simulink library "mlepLibrary"  (R2018a)
settings: Solver=ode45  StartTime=0.0  StopTime=10.0  RelTol=1e-3
undefined symbols (not defined in the file or in its folder): cs_val
settings Model: Creator=willyg  LastModifiedBy=E592090
settings DataIOCC: LimitDataPoints=on  SaveFormat=Array  SignalLoggingSaveFormat=ModelDataLogs
settings OptimizationCC: BlockReduction=off  BooleanDataType=off  LifeSpan=inf
settings DebuggingCC: SaveWithParameterizedLinksMsg=none  UnderspecifiedInitializationDetection=Classic  MergeDetectMultiDrivingBlocksExec=none  SignalResolutionControl=TryResolveAllWithWarning  MultiTaskDSMMsg=warning  MultiTaskCondExecSysMsg=none  SFUnexpectedBacktrackingDiag=warning  SFNoUnconditionalDefaultTransitionDiag=warning  SFExecutionAtInitializationDiag=none
settings HardwareCC: ProdBitPerPointer=32  ProdBitPerSizeT=32  ProdBitPerPtrDiffT=32  ProdLargestAtomicFloat=None  ProdIntDivRoundTo=Undefined  ProdEndianess=Unspecified  ProdWordSize=32  ProdHWDeviceType=32-bit Generic  TargetUnknown=on
settings ModelReferenceCC: PropagateSignalLabelsOutOfModel=off
settings CodeAppCC: StateflowObjectComments=on
settings GRTTargetCC: TargetLangStandard=C89/C90 (ANSI)  GeneratePreprocessorConditionals=Disable all
settings ConfigComp: CovMetricSettings=dw  CovHtmlReporting=on  CovSaveCumulativeToWorkspaceVar=on  CovSaveSingleToWorkspaceVar=on  CovExternalEMLEnable=off

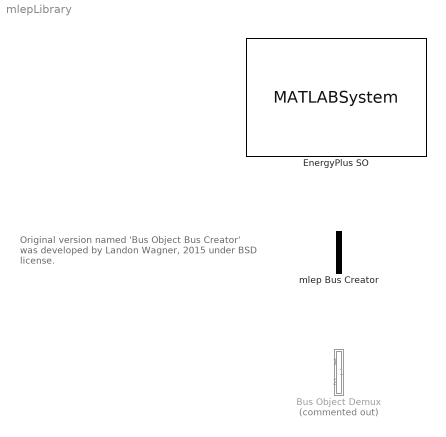
== system mlepLibrary ==
  note: Original version named 'Bus Object Bus Creator'
      | was developed by Landon Wagner, 2015 under
      | BSD license.
  Bus Object Demux : Subsystem  Commented=on  mask{busType=Bus: epInbus, bs_done=[]}
      mask prompts: busType "Bus Type"
      mask TypeOptions busType: Bus: epInbus | Bus: epOutbus
      mask Callback busType:
      | % Using variable names terminated with "_BOBC" to lessen the chances of
      | % collisions with existing workspace variables.
      | 
      | % Get the current block handle and mask handle.
      | handleCreator_BOBC = gcbh;
      | maskObj_BOBC       = Simulink.Mask.get(gcb);
      | 
      | % Get a list of variables in the workspace in order to search for the '1x1
      | % Bus' types.
      | wsVars_BOBC = whos;
      | 
      | % Reset the 'TypeOptions' bus list in case some '1x1 Bus' types have been
      | % deleted from or added to the workspace.
      | opts = {'<empty>'};
      | 
      | % Current number of options
      | old_opts = maskObj_BOBC.Parameters.TypeOptions;
      | 
      | % Reset the bus count.
      | busCount_BOBC = 0;
      | 
      | for index_BOBC = 1:length(wsVars_BOBC)
      | 
      |    % If the variable is a bus object...
      |    if strcmp(wsVars_BOBC(index_BOBC).class, 'Simulink.Bus')
      | 
      |       busCount_BOBC = busCount_BOBC + 1;
      | 
      |       % ... add it to the TypeOptions of the mask.
      |       opts(busCount_BOBC) = {['Bus: ', wsVars_BOBC(index_BOBC).name]};
      |    end
      | end
      | 
      | if busCount_BOBC == 0
      | 
      |    % If there are NO bus objects in the workspace then provide a warning
      |    % popup...
      |    %warning('There are currently no bus objects in the workspace - you have no use for this block. Use a normal Bus Creator instead.')
      | 
      |    % ... and do nothing.
      | % elseif ~strcmp(get_param(handleCreator_BOBC, 'OutDataTypeStr'), 'Inherit: auto')
      | %
      | %    % If the currently selected bus data type ('OutDataTypeStr') is not
      | %    % 'Inherit: auto' (i.e., if we are reopening the mask.) then get the
      | %    % current 'OutDataTypeStr' and 'maskVal.' ('maskVal' is the selected
      | %    % 'TypeOptions' list member.)
      | %    outDatStr_BOBC = get_param(handleCreator_BOBC, 'OutDataTypeStr');
      | %    maskVal_BOBC   = get_param(handleCreator_BOBC, 'MaskValues');
      | %
      | %    if ~strcmp(outDatStr_BOBC, maskVal_BOBC{1})
      | %
      | %       % Upon re-opening the mask if the default 'TypeOptions' list member
      | %       % (The first one.) contained in 'maskVal' does not match the
      | %       % currently selected bus data type ('OutDataTypeStr') then set the
      | %       % 'TypeOptions' list member to the selected bus data type. (Cuts down
      | %       % on confusion to have the displayed list member match the selected
      | %       % bus data type rather than the first entry.)
      | %       set_param(handleCreator_BOBC, 'MaskValues', {outDatStr_BOBC});
      | %    end
      | end
      | 
      | if ~strcmp([old_opts{:}],[opts{:}])
      |     maskObj_BOBC.Parameters.TypeOptions = opts;
      | end
      | 
      | % Clean up the workspace.
      | clear  handleCreator_BOBC  maskObj_BOBC     wsVars_BOBC ...
      |             busCount_BOBC    index_BOBC  outDatStr_BOBC ...
      |              maskVal_BOBC          opts        old_opts
      mask DialogControl applyMOCBSelection Prompt: Select signals
      mask DialogControl applyMOCBSelection Callback: run('clbk.m');
  EnergyPlus SO : MATLABSystem  System=mlepSO  idfFile=in.idf  epwFile=in.epw  SimulateUsing=Interpreted execution  useBus=on  inputBusName=epInbus  outputBusName=epOutbus
      mask Type: mlepSO
      mask Display:
      | image('mlepIcon.jpg');
      | port_label('input',1,'epInbus');
      | port_label('output',1,'epOutbus');
      | port_label('output',2,'Time');
      | port_label('output',3,'Flag');
  mlep Bus Creator : BusCreator  Inputs=1  mask(BUS OBJECT Bus Creator){busType=Bus: epInbus}
      mask prompts: busType "Bus Type"
      mask help:
      | Provides users the cabability to painlessly, instantly customize bus creators of output data type 'Bus:' by selecting the bus object type from a drop down menu dynamically populated by bus objects in the workspace.
      |
      | After pressing the "Apply Selection" button signal lines into the creator are populated and named with the elements in the chosen bus saving the user from having to recall and fill out signal line names.
      |
      | NOTE that when copying a Bus Object Bus Creator from your locked Library the link to the Library is automatically broken. This saves the user from having to Unlock Links To Library (From the Library menu.), Disable Link and finally Break Link (Both from the Model menu.) for every placed instance of the block.
      settings: AttributesFormatString=%<OutDataTypeStr>  CopyFcn=set_param(gcb, 'LinkStatus', 'none')
      mask TypeOptions busType: Bus: epInbus | Bus: epOutbus
      mask Callback busType:
      | % Using variable names terminated with "_BOBC" to lessen the chances of
      | % collisions with existing workspace variables.
      | 
      | % Get the current block handle and mask handle.
      | handleCreator_BOBC = gcbh;
      | maskObj_BOBC       = Simulink.Mask.get(gcb);
      | 
      | % Get a list of variables in the workspace in order to search for the '1x1
      | % Bus' types.
      | wsVars_BOBC = whos;
      | 
      | % Reset the 'TypeOptions' bus list in case some '1x1 Bus' types have been
      | % deleted from or added to the workspace.
      | opts = {'<empty>'};
      | 
      | % Current number of options
      | old_opts = maskObj_BOBC.Parameters.TypeOptions;
      | 
      | % Reset the bus count.
      | busCount_BOBC = 0;
      | 
      | for index_BOBC = 1:length(wsVars_BOBC)
      | 
      |    % If the variable is a bus object...
      |    if strcmp(wsVars_BOBC(index_BOBC).class, 'Simulink.Bus')
      | 
      |       busCount_BOBC = busCount_BOBC + 1;
      | 
      |       % ... add it to the TypeOptions of the mask.
      |       opts(busCount_BOBC) = {['Bus: ', wsVars_BOBC(index_BOBC).name]};
      |    end
      | end
      | 
      | if busCount_BOBC == 0
      | 
      |    % If there are NO bus objects in the workspace then provide a warning
      |    % popup...
      |    warning('There are currently no bus objects in the workspace - you have no use for this block. Use a normal Bus Creator instead.')
      | 
      |    % ... and do nothing.
      | elseif ~strcmp(get_param(handleCreator_BOBC, 'OutDataTypeStr'), 'Inherit: auto')
      | 
      |    % If the currently selected bus data type ('OutDataTypeStr') is not
      |    % 'Inherit: auto' (i.e., if we are reopening the mask.) then get the
      |    % current 'OutDataTypeStr' and 'maskVal.' ('maskVal' is the selected
      |    % 'TypeOptions' list member.)
      |    outDatStr_BOBC = get_param(handleCreator_BOBC, 'OutDataTypeStr');
      |    maskVal_BOBC   = get_param(handleCreator_BOBC, 'MaskValues');
      | 
      |    if ~strcmp(outDatStr_BOBC, maskVal_BOBC{1})
      | 
      |       % Upon re-opening the mask if the default 'TypeOptions' list member
      |       % (The first one.) contained in 'maskVal' does not match the
      |       % currently selected bus data type ('OutDataTypeStr') then set the
      |       % 'TypeOptions' list member to the selected bus data type. (Cuts down
      |       % on confusion to have the displayed list member match the selected
      |       % bus data type rather than the first entry.)
      |       set_param(handleCreator_BOBC, 'MaskValues', {outDatStr_BOBC});
      |    end
      | end
      | 
      | if ~strcmp([old_opts{:}],[opts{:}])
      |     maskObj_BOBC.Parameters.TypeOptions = opts;
      | end
      | 
      | % Clean up the workspace.
      | clear  handleCreator_BOBC  maskObj_BOBC     wsVars_BOBC ...
      |             busCount_BOBC    index_BOBC  outDatStr_BOBC ...
      |              maskVal_BOBC          opts        old_opts
      mask DialogControl applyMOCBSelection Prompt: Apply Selection
      mask DialogControl applyMOCBSelection Callback:
      | % Using variable names terminated with "_BOBC" to lessen the chances of
      | % collisions with existing workspace variables.
      | 
      | % Get the current block, current block handle and mask handle.
      | currentBlock_BOBC  = gcb;
      | handleCreator_BOBC = gcbh;
      | 
      | % Get the desired bus type...
      | desiredBusType_BOBC = get_param(handleCreator_BOBC, 'busType');
      | 
      | % ... and set the 'OutDataTypeStr' to it.
      | set_param(handleCreator_BOBC, 'OutDataTypeStr', desiredBusType_BOBC);
      | 
      | %% First delete any existing lines on the port.
      | % Get the line handles.
      | lh_BOBC = get_param(handleCreator_BOBC, 'LineHandles');
      | 
      | % If any lines exist (Non- -1 line handles.), delete them and start over.
      | if max(lh_BOBC.Inport > 0)
      | 
      |    for index_BOBC = 1:length(lh_BOBC.Inport)
      | 
      |       if lh_BOBC.Inport(index_BOBC) > 0
      | 
      |          delete_line(lh_BOBC.Inport(index_BOBC))
      |       end
      |    end
      | end
      | 
      | %% Then work on adding new lines.
      | 
      | % Get the block path for 'add_line' function.
      | blockPath_BOBC = get_param(handleCreator_BOBC, 'Parent');
      | 
      | % Get the newly selected bus type ('OutDataTypeStr')...
      | mocbBusType_BOBC = get_param(currentBlock_BOBC, 'OutDataTypeStr');
      | 
      | % ... and parse off "Bus: " so the string of the desired bus contained in
      | % 'OutDataTypeStr' matches the raw workspace bus names.
      | mocbBusType_BOBC = mocbBusType_BOBC(6:end);
      | 
      | % Then evaluate the string containing the workspace bus name which will
      | % load the desired bus parameters.
      | busParams_BOBC = eval(mocbBusType_BOBC);
      | 
      | % From the parameters grab the number of lines to add.
      | numLines_BOBC = length(busParams_BOBC.Elements);
      | 
      | % Set the number of inputs of the masked bus creator to the number of lines
      | % to add.
      | set_param(handleCreator_BOBC, 'Inputs', num2str(numLines_BOBC));
      | 
      | % Set heigh
      | sz = get_param(handleCreator_BOBC, 'Position');
      | y0 = sz(2) + (sz(4)-sz(2))/2; % vertical center
      | h  = max(sz(4)-sz(2), numLines_BOBC*10); % height
      | sz = [sz(1), ...
      |       y0 - h/2, ...
      |       sz(3), ...
      |       y0 + h/2];
      | set_param(handleCreator_BOBC, 'Position', sz);
      | clear y0 h sz
      | 
      | % Get (Inputs.) port handles so we can grab the positions of them.
      | ph_BOBC = get_param(handleCreator_BOBC, 'PortHandles');
      | 
      | % Get longest signal name to adjust the line lenght right
      | names_BOBC = {busParams_BOBC.Elements.Name};
      | 
      | for index_BOBC = 1:numLines_BOBC
      | 
      |    % Get the position of input port number 'index_BOBC'.
      |    portPos_BOBC = get_param(ph_BOBC.Inport(index_BOBC), 'Position');
      | 
      |    % Add a line from 50 pixels left of the port position to the port
      |    % position. (This must be done because it's the lines that get named,
      |    % not the port positions.)
      |    portLine_BOBC = add_line(blockPath_BOBC, ...
      |        [portPos_BOBC - [ceil(50/10/2*max(strlength(names_BOBC)))+10 0]; portPos_BOBC]);
      | 
      |    % Rename the new line to the bus 'index_BOBC-st/nd/rd/th' element name.
      |    set_param(portLine_BOBC, 'Name', busParams_BOBC.Elements(index_BOBC).Name)
      | end
      | 
      | %% Cleanup the workspace.
      | clear    currentBlock_BOBC  handleCreator_BOBC      index_BOBC ...
      |        desiredBusType_BOBC             lh_BOBC  blockPath_BOBC ...
      |           mocbBusType_BOBC      busParams_BOBC   numLines_BOBC ...
      |                    ph_BOBC        portPos_BOBC   portLine_BOBC ...
      |                 names_BOBC

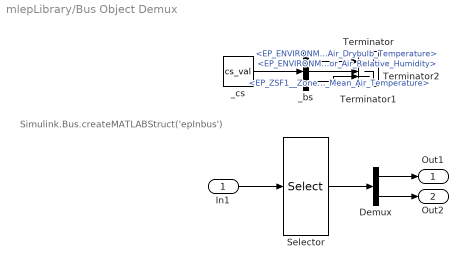
== system mlepLibrary/Bus Object Demux ==
  note: Simulink.Bus.createMATLABStruct('epInbus')
  In1 : Inport
  Demux : Demux  Outputs=2
  Selector : Selector  InputPortWidth=12  IndexOptions=Index vector (dialog)  Indices=[1 2]  OutputSizes=1
  Terminator : Terminator
  Terminator1 : Terminator
  Terminator2 : Terminator
  _bs : BusSelector  OutputSignals=EP_ENVIRONMENT__Site_Outdoor_Air_Drybulb_Temperature,EP_ENVIRONMENT__Site_Outdoor_Air_Relative_Humidity,EP_ZSF1__Zone_Mean_Air_Temperature
      mask init:
      | maskObj = Simulink.Mask.get(get_param(gcb,'Parent'));
      | maskObj.Initialization = '';
  _cs : Constant  Value=cs_val  OutDataTypeStr=Bus: epOutbus
  Out1 : Outport
  Out2 : Outport  Port=2
  wires:
  _cs/1 -> _bs/1
  In1/1 -> Selector/1
  Selector/1 -> Demux/1
  Demux/1 -> Out1/1
  Demux/2 -> Out2/1
  _bs/1 -> Terminator/1  "<EP_ENVIRONMENT__Site_Outdoor_Air_Drybulb_Temperature>"
  _bs/2 -> Terminator1/1  "<EP_ENVIRONMENT__Site_Outdoor_Air_Relative_Humidity>"
  _bs/3 -> Terminator2/1  "<EP_ZSF1__Zone_Mean_Air_Temperature>"
